simulink model "afe_abc_inv_psm_2mods"  (R2025b)
settings: Solver=ode1be  StartTime=0.0  StopTime=simlength  FixedStep=tc  MaxStep=tc
values from neighbouring files (symbols this model uses):
  n1 = 35    [voltage_islandmode_spectrum_analysis.m]    (also in voltage_spectrum_analysis.m)
undefined symbols (not defined in the file or in its folder): Adrso, afe_pwm_phase_shift_mod1, afe_pwm_phase_shift_mod2, Amplitude_U, Amplitude_V, Amplitude_W, Aresd, Bresd, Cresd, Crso, CTRPIFF_CLIP_RELEASE, dead_time_AFE, dead_time_INV, deepNEGeta, deepNEGxi, deepPOSxi, emf_fb_p, emf_fb_p_ccaller_1, emf_fb_p_ccaller_2, emf_p, emf_p_ccaller_1, emf_p_ccaller_2, end_time_LVRT, fPWM_AFE, fPWM_INV, g0_161Hz, g0_500Hz, g1_161Hz, g1_500Hz, i_grid_neg_eta_lim, i_grid_neg_eta_red_lim, i_grid_neg_xi_lim, i_grid_neg_xi_red_lim, i_grid_pos_eta_lim, i_grid_pos_eta_red_lim, ibez, id_lim, ieta_neg_ref_lim, ieta_pos_ref_lim, Igrid_phase_normalization_factor, inv_pwm_phase_shift_mod1, iq_lim, ixi_pos_ref_lim, k_frt_ref, kg, ki_afe, ki_i, ki_rc_neg_grid, ki_rc_pos_grid, ki_vs, ki_w, kp_afe, kp_i, kp_rc_neg_grid, kp_rc_pos_grid, kp_vs, kp_w, kw, l1, l2 ... (+55)
libraries: fl_lib x215, nesl_utility x107, simulink x22, cstblocks x18, threephase_inductor_lib x4, single_phase_transformer_lib x3, flexshaft_lib x1, psm x1
(part 10 of 17)

== system afe_abc_inv_psm_2mods/afe_abc_inv_psm_mod1/AFE_control/afe_control/grid_voltage_phase_lock_loops/dq_pll_ccaller/first_harmonic_tracker_phase_w ==
  u : Inport
  Bus Selector : BusSelector  OutputSignals=output_pu_hat
  C Caller : CCaller  FunctionName=first_harmonic_tracker_process_simulink  PortSpecificationStruct="%)30     .    V @   8    (     @         %    \"     4    !     0         %  0 \"0    $    _    07)G3F%M90  4&]R=$YA;64 4V-O<&4     26YD97@     5'EP90      4VEZ90      27-';&]B86P   X    P    !@    @    $          4    (     0    ,    !         !   P!O=70 #@   #     &    \"     0         !0    @    !     P    $         $  # &]U=  .    .     8    (    !          %    \"     $    &     0         0   ...(+2669 chars)"
  Constant : Constant  Value=ts_afe
  Constant1 : Constant  Value=4
  Data Type Conversion1 : DataTypeConversion  OutDataTypeStr=single  SaturateOnIntegerOverflow=off  RndMeth=Floor
  Data Type Conversion2 : DataTypeConversion  OutDataTypeStr=single  SaturateOnIntegerOverflow=off  RndMeth=Floor
  Data Type Conversion3 : DataTypeConversion  OutDataTypeStr=uint8  SaturateOnIntegerOverflow=off  RndMeth=Floor
  Data Type Conversion4 : DataTypeConversion  OutDataTypeStr=double  SaturateOnIntegerOverflow=off  RndMeth=Floor
  Data Type Conversion5 : DataTypeConversion  OutDataTypeStr=uint8  SaturateOnIntegerOverflow=off  RndMeth=Floor
  Step : Step  Time=0.0125  Before=1  After=0
  u_hat : Outport
  wires:
  Data Type Conversion4/1 -> u_hat/1
  Data Type Conversion3/1 -> C Caller/1
  Data Type Conversion1/1 -> C Caller/3
  Data Type Conversion2/1 -> C Caller/2
  C Caller/1 -> Bus Selector/1
  Bus Selector/1 -> Data Type Conversion4/1  "<output_pu_hat>"
  Step/1 -> Data Type Conversion3/1
  u/1 -> Data Type Conversion2/1
  Constant/1 -> Data Type Conversion1/1
  Data Type Conversion5/1 -> C Caller/4
  Constant1/1 -> Data Type Conversion5/1

== system afe_abc_inv_psm_2mods/afe_abc_inv_psm_mod1/AFE_control/afe_control/grid_voltage_sequences/voltage_sequence_avg/average_filter_ccaller ==
  v_grid_pos_xi : Inport
  v_grid_pos_eta : Inport  Port=2
  v_grid_neg_xi : Inport  Port=3
  v_grid_neg_eta : Inport  Port=4
  Moving Average Filter1 : Subsystem
  Moving Average Filter2 : Subsystem
  Moving Average Filter3 : Subsystem
  Moving Average Filter4 : Subsystem
  v_grid_pos_xi_avg : Outport
  v_grid_pos_eta_avg : Outport  Port=2
  v_grid_neg_xi_avg : Outport  Port=3
  v_grid_neg_eta_avg : Outport  Port=4
  wires:
  Moving Average Filter2/1(xi) -> v_grid_pos_eta_avg/1
  [omega_grid_pll_mod1] -> Moving Average Filter1/2(In3), Moving Average Filter2/2(In3), Moving Average Filter4/2(In3), Moving Average Filter3/2(In3)
  v_grid_pos_xi/1 -> Moving Average Filter1/1(In2)
  v_grid_neg_xi/1 -> Moving Average Filter3/1(In2)
  v_grid_neg_eta/1 -> Moving Average Filter4/1(In2)
  Moving Average Filter3/1(xi) -> v_grid_neg_xi_avg/1
  Moving Average Filter4/1(xi) -> v_grid_neg_eta_avg/1
  Moving Average Filter1/1(xi) -> v_grid_pos_xi_avg/1
  v_grid_pos_eta/1 -> Moving Average Filter2/1(In2)

== system afe_abc_inv_psm_2mods/afe_abc_inv_psm_mod1/AFE_control/afe_control/grid_voltage_sequences/voltage_sequence_avg/average_filter_simulink ==
  v_grid_pos_xi : Inport
  v_grid_pos_eta : Inport  Port=2
  v_grid_neg_xi : Inport  Port=3
  v_grid_neg_eta : Inport  Port=4
  moving_avarage_1 : Subsystem
  moving_avarage_2 : Subsystem
  moving_avarage_3 : Subsystem
  moving_avarage_4 : Subsystem
  v_grid_pos_xi_avg : Outport
  v_grid_pos_eta_avg : Outport  Port=2
  v_grid_neg_xi_avg : Outport  Port=3
  v_grid_neg_eta_avg : Outport  Port=4
  wires:
  v_grid_neg_xi/1 -> moving_avarage_3/1(u)
  v_grid_pos_xi/1 -> moving_avarage_1/1(u)
  v_grid_neg_eta/1 -> moving_avarage_4/1(u)
  v_grid_pos_eta/1 -> moving_avarage_2/1(u)
  moving_avarage_1/1(y) -> v_grid_pos_xi_avg/1  "v_grid_pos_xi_avg"
  moving_avarage_2/1(y) -> v_grid_pos_eta_avg/1  "v_grid_pos_eta_avg"
  moving_avarage_3/1(y) -> v_grid_neg_xi_avg/1  "v_grid_neg_xi_avg"
  moving_avarage_4/1(y) -> v_grid_neg_eta_avg/1  "v_grid_neg_eta_avg"

== system afe_abc_inv_psm_2mods/afe_abc_inv_psm_mod1/INV_control/inverter_control/current_ctrl/bemf_observer/bemf_observer ==
  ialpha_pu : Inport
  ibeta_pu : Inport  Port=2
  ualpha_pu : Inport  Port=3
  ubeta_pu : Inport  Port=4
  udc_pu : Inport  Port=5
  Gain : Gain  Gain=psi_m_norm
  Gain1 : Gain  Gain=psi_m_norm
  Trigonometric Function : Trigonometry  Operator=cos
  Trigonometric Function1 : Trigonometry
  double_integrator_observer : Subsystem
  psi_alpha_hat : Subsystem
  psi_beta_hat : Subsystem
  theta_bemf_hat : Subsystem
  omega_pu : Outport
  theta_hat : Outport  Port=2
  tag scope: psi_r_alpha_hat_mod1=global, psi_r_alpha_pu_hat_mod1=global, psi_r_beta_hat_mod1=global, psi_r_beta_pu_hat_mod1=global, psi_r_m_alpha_mod1=global, psi_r_m_beta_mod1=global, theta_bemf_hat_mod1=global
  wires:
  Trigonometric Function/1 -> Gain/1
  Trigonometric Function1/1 -> Gain1/1
  ialpha_pu/1 -> psi_alpha_hat/2(ialpha)
  ibeta_pu/1 -> psi_beta_hat/2(ibeta)
  psi_alpha_hat/2(psi_r_alpha_hat) -> [psi_r_alpha_hat_mod1]
  psi_beta_hat/2(psi_r_beta_hat) -> [psi_r_beta_hat_mod1]
  [psi_r_alpha_hat_mod1] -> theta_bemf_hat/1(psi_r_alpha_hat)
  [psi_r_beta_hat_mod1] -> theta_bemf_hat/2(psi_r_beta_hat)
  ualpha_pu/1 -> psi_alpha_hat/1(ualpha)
  ubeta_pu/1 -> psi_beta_hat/1(ubeta)
  [theta_hat_mod1] -> Trigonometric Function/1, Trigonometric Function1/1
  Gain/1 -> [psi_r_m_alpha_mod1]
  Gain1/1 -> [psi_r_m_beta_mod1]
  theta_bemf_hat/1(theta_emf_hat) -> [theta_bemf_hat_mod1]
  [theta_bemf_hat_mod1] -> double_integrator_observer/1(theta)
  double_integrator_observer/1(omega_pu_hat) -> omega_pu/1
  double_integrator_observer/2(theta_hat) -> theta_hat/1
  [psi_r_alpha_hat_mod1] -> [psi_r_alpha_pu_hat_mod1]
  [psi_r_beta_hat_mod1] -> [psi_r_beta_pu_hat_mod1]
  udc_pu/1 -> psi_beta_hat/3(udc), psi_alpha_hat/3(udc)

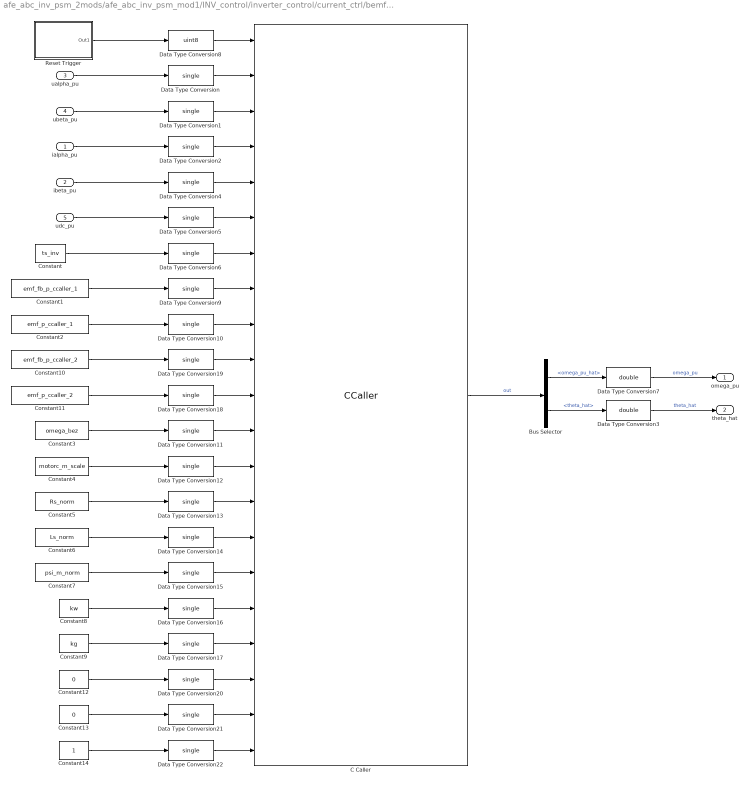
== system afe_abc_inv_psm_2mods/afe_abc_inv_psm_mod1/INV_control/inverter_control/current_ctrl/bemf_observer/bemf_observer_ccaller ==
  ialpha_pu : Inport
  ibeta_pu : Inport  Port=2
  ualpha_pu : Inport  Port=3
  ubeta_pu : Inport  Port=4
  udc_pu : Inport  Port=5
  Bus Selector : BusSelector  OutputSignals=omega_pu_hat,theta_hat
  C Caller : CCaller  FunctionName=bemf_obsv_process_simulink  PortSpecificationStruct="%)30     .    N\"8   8    (     @         %    \"    !8    !     0         %  0 \"0    $    _    07)G3F%M90  4&]R=$YA;64 4V-O<&4     26YD97@     5'EP90      4VEZ90      27-';&]B86P   X    P    !@    @    $          4    (     0    ,    !         !   P!O=70 #@   #     &    \"     0         !0    @    !     P    $         $  # &]U=  .    .     8    (    !          %    \"     $    &     0         0  ...(+12985 chars)"
  Constant : Constant  Value=ts_inv
  Constant1 : Constant  Value=emf_fb_p_ccaller_1
  Constant10 : Constant  Value=emf_fb_p_ccaller_2
  Constant11 : Constant  Value=emf_p_ccaller_2
  Constant12 : Constant  Value=0
  Constant13 : Constant  Value=0
  Constant14 : Constant
  Constant2 : Constant  Value=emf_p_ccaller_1
  Constant3 : Constant  Value=omega_bez
  Constant4 : Constant  Value=motorc_m_scale
  Constant5 : Constant  Value=Rs_norm
  Constant6 : Constant  Value=Ls_norm
  Constant7 : Constant  Value=psi_m_norm
  Constant8 : Constant  Value=kw
  Constant9 : Constant  Value=kg
  Data Type Conversion{,1..2,4..6,9..22} (20 alike) : DataTypeConversion  OutDataTypeStr=single  SaturateOnIntegerOverflow=off  RndMeth=Floor
  Data Type Conversion3 : DataTypeConversion  OutDataTypeStr=double  SaturateOnIntegerOverflow=off  RndMeth=Floor
  Data Type Conversion7 : DataTypeConversion  OutDataTypeStr=double  SaturateOnIntegerOverflow=off  RndMeth=Floor
  Data Type Conversion8 : DataTypeConversion  OutDataTypeStr=uint8  SaturateOnIntegerOverflow=off  RndMeth=Floor
  Reset Trigger : Subsystem
  omega_pu : Outport
  theta_hat : Outport  Port=2
  wires:
  Data Type Conversion5/1 -> C Caller/6
  Data Type Conversion/1 -> C Caller/2
  C Caller/1 -> Bus Selector/1  "out"
  Data Type Conversion1/1 -> C Caller/3
  Data Type Conversion4/1 -> C Caller/5
  Data Type Conversion2/1 -> C Caller/4
  Data Type Conversion6/1 -> C Caller/7
  Bus Selector/2 -> Data Type Conversion3/1  "<theta_hat>"
  Bus Selector/1 -> Data Type Conversion7/1  "<omega_pu_hat>"
  Data Type Conversion7/1 -> omega_pu/1  "omega_pu"
  Data Type Conversion3/1 -> theta_hat/1  "theta_hat"
  Data Type Conversion8/1 -> C Caller/1
  Data Type Conversion9/1 -> C Caller/8
  Data Type Conversion10/1 -> C Caller/9
  Data Type Conversion19/1 -> C Caller/10
  Data Type Conversion18/1 -> C Caller/11
  Data Type Conversion11/1 -> C Caller/12
  Data Type Conversion12/1 -> C Caller/13
  Data Type Conversion13/1 -> C Caller/14
  Data Type Conversion14/1 -> C Caller/15
  Data Type Conversion15/1 -> C Caller/16
  Data Type Conversion16/1 -> C Caller/17
  Data Type Conversion17/1 -> C Caller/18
  Data Type Conversion20/1 -> C Caller/19
  Data Type Conversion21/1 -> C Caller/20
  Data Type Conversion22/1 -> C Caller/21
  Constant14/1 -> Data Type Conversion22/1
  Constant13/1 -> Data Type Conversion21/1
  Constant12/1 -> Data Type Conversion20/1
  Constant9/1 -> Data Type Conversion17/1
  Constant8/1 -> Data Type Conversion16/1
  Constant7/1 -> Data Type Conversion15/1
  Constant6/1 -> Data Type Conversion14/1
  Constant5/1 -> Data Type Conversion13/1
  Constant4/1 -> Data Type Conversion12/1
  Constant3/1 -> Data Type Conversion11/1
  Constant11/1 -> Data Type Conversion18/1
  Constant10/1 -> Data Type Conversion19/1
  Constant2/1 -> Data Type Conversion10/1
  Constant1/1 -> Data Type Conversion9/1
  Constant/1 -> Data Type Conversion6/1
  ibeta_pu/1 -> Data Type Conversion4/1
  ialpha_pu/1 -> Data Type Conversion2/1
  ubeta_pu/1 -> Data Type Conversion1/1
  ualpha_pu/1 -> Data Type Conversion/1
  Reset Trigger/1(Out1) -> Data Type Conversion8/1
  udc_pu/1 -> Data Type Conversion5/1

== system afe_abc_inv_psm_2mods/afe_abc_inv_psm_mod1/INV_control/inverter_control/current_ctrl/bemf_observer/phase_fault ==
  double_integrator_observer : Subsystem
  phase_fault : Subsystem
  omega_pu_encoder : Outport
  theta_hat_encoder : Outport  Port=2
  wires:
  [theta_elec_psm] -> phase_fault/1(theta_pmsm)  "theta_pmsm"
  double_integrator_observer/2(theta_hat) -> theta_hat_encoder/1  "theta_hat_encoder"
  phase_fault/1(theta) -> double_integrator_observer/1(theta)
  double_integrator_observer/1(omega_pu_hat) -> omega_pu_encoder/1  "omega_pu_encoder"

== system afe_abc_inv_psm_2mods/afe_abc_inv_psm_mod1/INV_control/inverter_control/current_ctrl/current_ctrl/MTPA _mod1 ==
  iq_ref : Inport
  Gain1 : Gain  Gain=1/(Ld_norm - Lq_norm)/2
  Gain2 : Gain  Gain=1/(Ld_norm - Lq_norm)/2
  Gain3 : Gain  Gain=-1
  Math Function1 : Math  Operator=magnitude^2  SignedPower=on
  Math Function4 : Math  Operator=magnitude^2  SignedPower=on
  Sqrt : Sqrt
  Sum : Sum  Inputs=|++
  Sum1 : Sum  Inputs=|-+
  id_ref_pu < x < 0 : Saturate  UpperLimit=0  LowerLimit=-id_lim
  Id_ref_mtpa : Outport  VectorParamsAs1DForOutWhenUnconnected=off
  wires:
  Sum1/1 -> Gain3/1
  id_ref_pu < x < 0/1 -> Id_ref_mtpa/1
  Math Function4/1 -> Sum/1
  Math Function1/1 -> Sum/2
  Gain1/1 -> Math Function4/1
  Sum/1 -> Sqrt/1
  Sqrt/1 -> Sum1/2
  iq_ref/1 -> Math Function1/1
  Gain2/1 -> Sum1/1
  [omega_hat_pu_mod1] -> Gain1/1, Gain2/1
  Gain3/1 -> id_ref_pu < x < 0/1

== system afe_abc_inv_psm_2mods/afe_abc_inv_psm_mod1/INV_control/inverter_control/current_ctrl/current_ctrl/dq_pi_with_vector_antiwindup mod1 ==
  id_ref : Inport
  id : Inport  Port=2
  iq_ref : Inport  Port=3
  iq : Inport  Port=4
  udc_pu : Inport  Port=5
  Variant Source : VariantSource  VariantControls={use_current_controller_from_simulink_module_1 == 1, use_current_controller_from_ccaller_module_1 == 1}
  Variant Source1 : VariantSource  VariantControls={use_current_controller_from_simulink_module_1 == 1, use_current_controller_from_ccaller_module_1 == 1}
  dq_vector_pi : Subsystem
  dq_vector_pi_ccaller : Subsystem
  simulink/Ccaller VectorPI : Scope  NumInputPorts=2
      settings: ActiveDisplayYMinimum=-0.12579688616096973  ActiveDisplayYMaximum=0.43534495122730732
  ctrl_d_u : Outport
  ctrl_q_u : Outport  Port=2
  wires:
  id/1 -> dq_vector_pi_ccaller/1(id), dq_vector_pi/1(id)  "id"
  id_ref/1 -> dq_vector_pi_ccaller/2(id_ref), dq_vector_pi/2(id_ref)  "id_ref"
  iq/1 -> dq_vector_pi_ccaller/3(iq), dq_vector_pi/3(iq)  "iq"
  iq_ref/1 -> dq_vector_pi_ccaller/4(iq_ref), dq_vector_pi/4(iq_ref)  "iq_ref"
  dq_vector_pi/1(md_sat) -> Variant Source/1
  dq_vector_pi_ccaller/2(uq_ctrl_out) -> Variant Source1/2
  dq_vector_pi/2(mq_sat) -> Variant Source1/1
  dq_vector_pi_ccaller/1(ud_ctrl_out) -> Variant Source/2
  Variant Source/1 -> ctrl_d_u/1, simulink/Ccaller VectorPI/1  "ctrl_d_u"
  Variant Source1/1 -> simulink/Ccaller VectorPI/2, ctrl_q_u/1  "ctrl_q_u"
  udc_pu/1 -> dq_vector_pi_ccaller/5(udc_pu)

== system afe_abc_inv_psm_2mods/afe_abc_inv_psm_mod1/INV_control/inverter_control/current_ctrl/current_ctrl/id_ref _mod1 ==
  id_mtpa : Inport
  Constant : Constant  Value=0
  Variant Source : VariantSource  VariantControls={use_mtpa == 1, use_mtpa == 0}
  id_ref : Outport
  wires:
  Variant Source/1 -> id_ref/1
  id_mtpa/1 -> Variant Source/1
  Constant/1 -> Variant Source/2

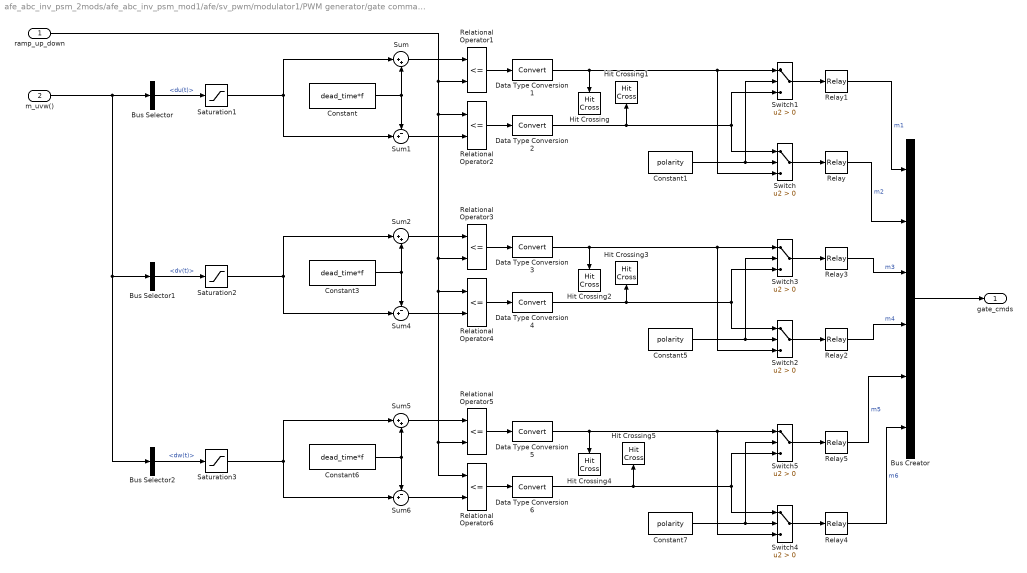
== system afe_abc_inv_psm_2mods/afe_abc_inv_psm_mod1/afe/sv_pwm/modulator1/PWM generator/gate commands ==
  ramp_up_down : Inport
  m_uvw() : Inport  Port=2
  Bus Creator : BusCreator  Inputs=6
  Bus Selector : BusSelector  OutputSignals=du(t)
  Bus Selector1 : BusSelector  OutputSignals=dv(t)
  Bus Selector2 : BusSelector  OutputSignals=dw(t)
  Constant : Constant  Value=dead_time*f
  Constant1 : Constant  Value=polarity
  Constant3 : Constant  Value=dead_time*f
  Constant5 : Constant  Value=polarity
  Constant6 : Constant  Value=dead_time*f
  Constant7 : Constant  Value=polarity
  Data Type Conversion{1..6} (6 alike) : DataTypeConversion
  Hit Crossing{,1..5} (6 alike) : HitCross  ShowOutputPort=off
  Relational Operator{1..6} (6 alike) : RelationalOperator  Operator=<=  InputSameDT=off
  Relay{,1..5} (6 alike) : Relay  OnOutputValue=pos_cmd_gate  OffOutputValue=neg_cmd_gate
  Saturation1 : Saturate  UpperLimit=m_up  LowerLimit=m_low
  Saturation2 : Saturate  UpperLimit=m_up  LowerLimit=m_low
  Saturation3 : Saturate  UpperLimit=m_up  LowerLimit=m_low
  Sum : Sum  Inputs=|++  SaturateOnIntegerOverflow=on
  Sum1 : Sum  Inputs=-+|  SaturateOnIntegerOverflow=on
  Sum2 : Sum  Inputs=|++  SaturateOnIntegerOverflow=on
  Sum4 : Sum  Inputs=-+|  SaturateOnIntegerOverflow=on
  Sum5 : Sum  Inputs=|++  SaturateOnIntegerOverflow=on
  Sum6 : Sum  Inputs=-+|  SaturateOnIntegerOverflow=on
  Switch{,1..5} (6 alike) : Switch  Criteria=u2 > Threshold  SaturateOnIntegerOverflow=off  InputSameDT=off
  gate_cmds : Outport
  wires:
  Data Type Conversion6/1 -> Switch4/1, Switch5/3, Hit Crossing5/1
  Constant1/1 -> Switch1/2, Switch/2
  Data Type Conversion1/1 -> Switch/3, Switch1/1, Hit Crossing/1
  Constant3/1 -> Sum4/1, Sum2/2
  m_uvw()/1 -> Bus Selector2/1, Bus Selector1/1, Bus Selector/1
  Relay4/1 -> Bus Creator/6  "m6"
  Constant6/1 -> Sum5/2, Sum6/1
  Saturation1/1 -> Sum1/2, Sum/1
  Data Type Conversion3/1 -> Switch2/3, Switch3/1, Hit Crossing2/1
  Data Type Conversion2/1 -> Switch/1, Switch1/3, Hit Crossing1/1
  Relational Operator1/1 -> Data Type Conversion1/1
  Bus Creator/1 -> gate_cmds/1
  Data Type Conversion5/1 -> Switch4/3, Switch5/1, Hit Crossing4/1
  Sum1/1 -> Relational Operator2/2
  Constant5/1 -> Switch2/2, Switch3/2
  Switch/1 -> Relay/1
  Sum/1 -> Relational Operator1/1
  Relational Operator6/1 -> Data Type Conversion6/1
  Relay2/1 -> Bus Creator/4  "m4"
  Saturation3/1 -> Sum5/1, Sum6/2
  Constant7/1 -> Switch5/2, Switch4/2
  Sum5/1 -> Relational Operator5/1
  Bus Selector/1 -> Saturation1/1  "<du(t)>"
  Data Type Conversion4/1 -> Switch2/1, Switch3/3, Hit Crossing3/1
  ramp_up_down/1 -> Relational Operator3/2, Relational Operator6/1, Relational Operator5/2, Relational Operator4/1, Relational Operator2/1, Relational Operator1/2
  Switch4/1 -> Relay4/1
  Relational Operator5/1 -> Data Type Conversion5/1
  Switch5/1 -> Relay5/1
  Saturation2/1 -> Sum4/2, Sum2/1
  Relational Operator3/1 -> Data Type Conversion3/1
  Sum2/1 -> Relational Operator3/1
  Switch1/1 -> Relay1/1
  Relay3/1 -> Bus Creator/3  "m3"
  Relational Operator2/1 -> Data Type Conversion2/1
  Bus Selector1/1 -> Saturation2/1  "<dv(t)>"
  Switch3/1 -> Relay3/1
  Sum4/1 -> Relational Operator4/2
  Relay/1 -> Bus Creator/2  "m2"
  Relational Operator4/1 -> Data Type Conversion4/1
  Bus Selector2/1 -> Saturation3/1  "<dw(t)>"
  Relay1/1 -> Bus Creator/1  "m1"
  Sum6/1 -> Relational Operator6/2
  Constant/1 -> Sum/2, Sum1/1
  Relay5/1 -> Bus Creator/5  "m5"
  Switch2/1 -> Relay2/1

== system afe_abc_inv_psm_2mods/afe_abc_inv_psm_mod1/inverter/inverter/sv_pwm/modulator1/PWM generator ==
  time_source : Inport
  phase : Inport  Port=2
  m_uvw() : Inport  Port=3
  Constant8 : Constant  Value=tc
  Constant9 : Constant  Value=f
  MATLAB Function : MATLAB Function  TreatAsAtomicUnit=on  SystemSampleTime=tc
  MATLAB Function1 : MATLAB Function  TreatAsAtomicUnit=on  SystemSampleTime=tc
  gate commands : Subsystem
  period : Constant  Value=1/f
  trgo : Outport
  gate_cmds : Outport  Port=2
  wires:
  period/1 -> MATLAB Function/3(period)
  phase/1 -> MATLAB Function/2(phase)
  MATLAB Function/1(y) -> gate commands/1(ramp_up_down), MATLAB Function1/3(ramp_up_down)
  MATLAB Function1/1(trgo) -> trgo/1
  Constant8/1 -> MATLAB Function1/1(sampling_time)
  Constant9/1 -> MATLAB Function1/2(fPWM)
  m_uvw()/1 -> gate commands/2(m_uvw())
  gate commands/1(gate_cmds) -> gate_cmds/1
  time_source/1 -> MATLAB Function/1(t)

== system afe_abc_inv_psm_2mods/afe_abc_inv_psm_mod2/AFE_control/afe_control/FRT-VDE4110/FRT-Detection/dvxi_n//dt ==
  x : Inport
  Gain : Gain  Gain=l1
  Gain1 : Gain  Gain=l2
  Gain5 : Gain  Gain=ts_afe
  Sum : Sum  Inputs=-+|
  Sum1 : Sum  Inputs=|++
  Sum2 : Sum  Inputs=|++
  Sum8 : Sum  Inputs=++|
  Unit Delay1 : UnitDelay  SampleTime=-1  HasFrameUpgradeWarning=on
  Unit Delay2 : UnitDelay  SampleTime=-1  HasFrameUpgradeWarning=on
  xdot_hat : Outport  VectorParamsAs1DForOutWhenUnconnected=off
  wires:
  Gain1/1 -> Sum2/1
  x/1 -> Sum/2  "x"
  Gain5/1 -> Sum8/1
  Sum1/1 -> Unit Delay2/1
  Gain/1 -> Sum1/1
  Unit Delay2/1 -> xdot_hat/1, Sum1/2, Gain5/1
  Sum2/1 -> Sum8/2
  Unit Delay1/1 -> Sum2/2, Sum/1  "x_hat"
  Sum/1 -> Gain1/1, Gain/1
  Sum8/1 -> Unit Delay1/1

== system afe_abc_inv_psm_2mods/afe_abc_inv_psm_mod2/AFE_control/afe_control/FRT-VDE4110/FRT-Detection/dvxi_p//dt ==
  x : Inport
  Gain : Gain  Gain=l1
  Gain1 : Gain  Gain=l2
  Gain5 : Gain  Gain=ts_afe
  Sum : Sum  Inputs=-+|
  Sum1 : Sum  Inputs=|++
  Sum2 : Sum  Inputs=|++
  Sum8 : Sum  Inputs=++|
  Unit Delay1 : UnitDelay  SampleTime=-1  HasFrameUpgradeWarning=on
  Unit Delay2 : UnitDelay  SampleTime=-1  HasFrameUpgradeWarning=on
  xdot_hat : Outport  VectorParamsAs1DForOutWhenUnconnected=off
  wires:
  Unit Delay2/1 -> Gain5/1, Sum1/2, xdot_hat/1
  Sum8/1 -> Unit Delay1/1
  Sum/1 -> Gain/1, Gain1/1
  Unit Delay1/1 -> Sum/1, Sum2/2  "x_hat"
  Sum2/1 -> Sum8/2
  Gain/1 -> Sum1/1
  Sum1/1 -> Unit Delay2/1
  Gain5/1 -> Sum8/1
  x/1 -> Sum/2  "x"
  Gain1/1 -> Sum2/1

== system afe_abc_inv_psm_2mods/afe_abc_inv_psm_mod2/AFE_control/afe_control/FRT-VDE4110/FRT-PosNegReactiveCurrentReferences/avg_flt_500ms ==
  In1 : Inport
  Constant : Constant  Value=2*pi/500e-3
  Constant1 : Constant  Value=ts_afe
  Constant2 : Constant
  Sum : Sum  Inputs=|-+
  avg_flt_1 : MATLAB Function  TreatAsAtomicUnit=on
  Out1 : Outport  VectorParamsAs1DForOutWhenUnconnected=off
  wires:
  Sum/1 -> avg_flt_1/4(enable)
  [frt_active_mod2] -> Sum/1
  Constant2/1 -> Sum/2
  In1/1 -> avg_flt_1/1(x)  "input"
  Constant/1 -> avg_flt_1/2(w)
  Constant1/1 -> avg_flt_1/3(ts)
  avg_flt_1/1(y1) -> Out1/1  "output"

== system afe_abc_inv_psm_2mods/afe_abc_inv_psm_mod2/AFE_control/afe_control/FRT-VDE4110/FRT-PosNegReactiveCurrentReferences/avg_flt_500ms1 ==
  In1 : Inport
  Constant : Constant  Value=2*pi/500e-3
  Constant1 : Constant  Value=ts_afe
  Constant2 : Constant
  Sum : Sum  Inputs=|-+
  avg_flt_1 : MATLAB Function  TreatAsAtomicUnit=on
  Out1 : Outport  VectorParamsAs1DForOutWhenUnconnected=off
  wires:
  avg_flt_1/1(y1) -> Out1/1  "output"
  Constant1/1 -> avg_flt_1/3(ts)
  Constant/1 -> avg_flt_1/2(w)
  In1/1 -> avg_flt_1/1(x)  "input"
  Constant2/1 -> Sum/2
  [frt_active_mod2] -> Sum/1
  Sum/1 -> avg_flt_1/4(enable)

== system afe_abc_inv_psm_2mods/afe_abc_inv_psm_mod2/AFE_control/afe_control/FRT-VDE4110/FRT-PosNegReactiveCurrentReferences/avg_flt_500ms2 ==
  In1 : Inport
  Constant : Constant  Value=2*pi/500e-3
  Constant1 : Constant  Value=ts_afe
  Constant2 : Constant
  Sum : Sum  Inputs=|-+
  avg_flt_1 : MATLAB Function  TreatAsAtomicUnit=on
  Out1 : Outport  VectorParamsAs1DForOutWhenUnconnected=off
  wires:
  Sum/1 -> avg_flt_1/4(enable)
  [frt_active_mod2] -> Sum/1
  Constant2/1 -> Sum/2
  In1/1 -> avg_flt_1/1(x)  "input"
  Constant/1 -> avg_flt_1/2(w)
  Constant1/1 -> avg_flt_1/3(ts)
  avg_flt_1/1(y1) -> Out1/1  "output"

== system afe_abc_inv_psm_2mods/afe_abc_inv_psm_mod2/AFE_control/afe_control/FRT-VDE4110/FRT-PosNegReactiveCurrentReferences/avg_flt_500ms3 ==
  In1 : Inport
  Constant : Constant  Value=2*pi/500e-3
  Constant1 : Constant  Value=ts_afe
  Constant2 : Constant
  Sum : Sum  Inputs=|-+
  avg_flt_1 : MATLAB Function  TreatAsAtomicUnit=on
  Out1 : Outport  VectorParamsAs1DForOutWhenUnconnected=off
  wires:
  avg_flt_1/1(y1) -> Out1/1  "output"
  Constant1/1 -> avg_flt_1/3(ts)
  Constant/1 -> avg_flt_1/2(w)
  In1/1 -> avg_flt_1/1(x)  "input"
  Constant2/1 -> Sum/2
  [frt_active_mod2] -> Sum/1
  Sum/1 -> avg_flt_1/4(enable)

== system afe_abc_inv_psm_2mods/afe_abc_inv_psm_mod2/AFE_control/afe_control/FRT-VDE4110/FRT-PosNegReactiveCurrentReferences/u_161Hz_flt1 ==
  input : Inport
  Gain3 : Gain  Gain=g1_161Hz
  Gain6 : Gain  Gain=g0_161Hz
  Sum : Sum  Inputs=|++
  Unit Delay1 : UnitDelay  SampleTime=-1  HasFrameUpgradeWarning=on
  output : Outport  VectorParamsAs1DForOutWhenUnconnected=off
  wires:
  Sum/1 -> output/1, Unit Delay1/1
  Gain3/1 -> Sum/2
  Unit Delay1/1 -> Gain3/1
  input/1 -> Gain6/1
  Gain6/1 -> Sum/1

== system afe_abc_inv_psm_2mods/afe_abc_inv_psm_mod2/AFE_control/afe_control/FRT-VDE4110/FRT-PosNegReactiveCurrentReferences/u_161Hz_flt2 ==
  input : Inport
  Gain3 : Gain  Gain=g1_161Hz
  Gain6 : Gain  Gain=g0_161Hz
  Sum : Sum  Inputs=|++
  Unit Delay1 : UnitDelay  SampleTime=-1  HasFrameUpgradeWarning=on
  output : Outport  VectorParamsAs1DForOutWhenUnconnected=off
  wires:
  Gain6/1 -> Sum/1
  input/1 -> Gain6/1
  Unit Delay1/1 -> Gain3/1
  Gain3/1 -> Sum/2
  Sum/1 -> Unit Delay1/1, output/1

== system afe_abc_inv_psm_2mods/afe_abc_inv_psm_mod2/AFE_control/afe_control/FRT-VDE4110/FRT-PosNegReactiveCurrentReferences/u_161Hz_flt3 ==
  input : Inport
  Gain3 : Gain  Gain=g1_161Hz
  Gain6 : Gain  Gain=g0_161Hz
  Sum : Sum  Inputs=|++
  Unit Delay1 : UnitDelay  SampleTime=-1  HasFrameUpgradeWarning=on
  output : Outport  VectorParamsAs1DForOutWhenUnconnected=off
  wires:
  Sum/1 -> output/1, Unit Delay1/1
  Gain3/1 -> Sum/2
  Unit Delay1/1 -> Gain3/1
  input/1 -> Gain6/1
  Gain6/1 -> Sum/1

== system afe_abc_inv_psm_2mods/afe_abc_inv_psm_mod2/AFE_control/afe_control/current_ctrl/Inner Loop Current Control/Current-Control, Phase a ==
  In1 : Inport
  In2 : Inport  Port=2
  Add : Sum
  Cresd./Tcontrol new1 : Gain  Gain=Cresd  Multiplication=Matrix(K*u)
  Gain : Gain  Gain=kp_afe
  Gain1 : Gain  Gain=ki_afe
  Gain2 : Gain  Gain=Bresd  Multiplication=Matrix(K*u)
  Gain3 : Gain  Gain=Aresd  Multiplication=Matrix(K*u)
  Sum : Sum  Inputs=|+-
  Sum2 : Sum  Inputs=|++  SaturateOnIntegerOverflow=on
  Unit Delay : UnitDelay  InitialCondition=[0 0]  SampleTime=-1  HasFrameUpgradeWarning=on
  Out1 : Outport
  wires:
  Cresd./Tcontrol new1/1 -> Add/2  "y(k)"
  Gain3/1 -> Sum2/2
  Sum2/1 -> Unit Delay/1  "x(k+1)"
  Unit Delay/1 -> Cresd./Tcontrol new1/1, Gain3/1  "x(k)"
  Gain2/1 -> Sum2/1
  Gain1/1 -> Gain2/1  "u(k)"
  Gain/1 -> Add/1
  Sum/1 -> Gain/1, Gain1/1
  Add/1 -> Out1/1  "v_a"
  In2/1 -> Sum/2  "isa"
  In1/1 -> Sum/1  "isa_ref"

== system afe_abc_inv_psm_2mods/afe_abc_inv_psm_mod2/AFE_control/afe_control/current_ctrl/Inner Loop Current Control/Current-Control, Phase b ==
  In1 : Inport
  In2 : Inport  Port=2
  Add : Sum
  Cresd./Tcontrol new1 : Gain  Gain=Cresd  Multiplication=Matrix(K*u)
  Gain : Gain  Gain=kp_afe
  Gain1 : Gain  Gain=ki_afe
  Gain2 : Gain  Gain=Bresd  Multiplication=Matrix(K*u)
  Gain3 : Gain  Gain=Aresd  Multiplication=Matrix(K*u)
  Sum : Sum  Inputs=|+-
  Sum2 : Sum  Inputs=|++  SaturateOnIntegerOverflow=on
  Unit Delay : UnitDelay  InitialCondition=[0 0]  SampleTime=-1  HasFrameUpgradeWarning=on
  Out1 : Outport
  wires:
  In1/1 -> Sum/1  "isb_ref"
  In2/1 -> Sum/2  "isb"
  Add/1 -> Out1/1  "v_a"
  Sum/1 -> Gain1/1, Gain/1
  Gain/1 -> Add/1
  Gain1/1 -> Gain2/1  "u(k)"
  Gain2/1 -> Sum2/1
  Unit Delay/1 -> Gain3/1, Cresd./Tcontrol new1/1  "x(k)"
  Sum2/1 -> Unit Delay/1  "x(k+1)"
  Gain3/1 -> Sum2/2
  Cresd./Tcontrol new1/1 -> Add/2  "y(k)"

== system afe_abc_inv_psm_2mods/afe_abc_inv_psm_mod2/AFE_control/afe_control/current_ctrl/Inner Loop Current Control/Current-Control, Phase c ==
  In1 : Inport
  In2 : Inport  Port=2
  Add : Sum
  Cresd./Tcontrol new1 : Gain  Gain=Cresd  Multiplication=Matrix(K*u)
  Gain : Gain  Gain=kp_afe
  Gain1 : Gain  Gain=ki_afe
  Gain2 : Gain  Gain=Bresd  Multiplication=Matrix(K*u)
  Gain3 : Gain  Gain=Aresd  Multiplication=Matrix(K*u)
  Sum : Sum  Inputs=|+-
  Sum2 : Sum  Inputs=|++  SaturateOnIntegerOverflow=on
  Unit Delay : UnitDelay  InitialCondition=[0 0]  SampleTime=-1  HasFrameUpgradeWarning=on
  Out1 : Outport
  wires:
  Cresd./Tcontrol new1/1 -> Add/2  "y(k)"
  Gain3/1 -> Sum2/2
  Sum2/1 -> Unit Delay/1  "x(k+1)"
  Unit Delay/1 -> Cresd./Tcontrol new1/1, Gain3/1  "x(k)"
  Gain2/1 -> Sum2/1
  Gain1/1 -> Gain2/1  "u(k)"
  Gain/1 -> Add/1
  Sum/1 -> Gain/1, Gain1/1
  Add/1 -> Out1/1  "v_a"
  In2/1 -> Sum/2  "isc"
  In1/1 -> Sum/1  "isc_ref"

== system afe_abc_inv_psm_2mods/afe_abc_inv_psm_mod2/AFE_control/afe_control/grid_current_sequences_and_reactive_pwr_ctrl/current_sequence_avg/average_filter_ccaller ==
  i_grid_pos_xi : Inport
  i_grid_pos_eta : Inport  Port=2
  i_grid_neg_xi : Inport  Port=3
  i_grid_neg_eta : Inport  Port=4
  Moving Average Filter1 : Subsystem
  Moving Average Filter2 : Subsystem
  Moving Average Filter3 : Subsystem
  Moving Average Filter5 : Subsystem
  i_grid_pos_xi_avg : Outport
  i_grid_pos_eta_avg : Outport  Port=2
  i_grid_neg_xi_avg : Outport  Port=3
  i_grid_neg_eta_avg : Outport  Port=4
  wires:
  Moving Average Filter5/1(xi) -> i_grid_pos_xi_avg/1
  i_grid_neg_eta/1 -> Moving Average Filter3/1(In2)
  i_grid_pos_xi/1 -> Moving Average Filter5/1(In2)
  Moving Average Filter2/1(xi) -> i_grid_neg_xi_avg/1
  i_grid_neg_xi/1 -> Moving Average Filter2/1(In2)
  Moving Average Filter3/1(xi) -> i_grid_neg_eta_avg/1
  i_grid_pos_eta/1 -> Moving Average Filter1/1(In2)
  [omega_grid_pll_mod2] -> Moving Average Filter2/2(In3), Moving Average Filter3/2(In3), Moving Average Filter1/2(In3), Moving Average Filter5/2(In3)
  Moving Average Filter1/1(xi) -> i_grid_pos_eta_avg/1

== system afe_abc_inv_psm_2mods/afe_abc_inv_psm_mod2/AFE_control/afe_control/grid_current_sequences_and_reactive_pwr_ctrl/current_sequence_avg/average_filter_simulink ==
  i_grid_pos_xi : Inport
  i_grid_pos_eta : Inport  Port=2
  i_grid_neg_xi : Inport  Port=3
  i_grid_neg_eta : Inport  Port=4
  moving_avarage_1 : Subsystem
  moving_avarage_2 : Subsystem
  moving_avarage_3 : Subsystem
  moving_avarage_4 : Subsystem
  i_grid_pos_xi_avg : Outport
  i_grid_pos_eta_avg : Outport  Port=2
  i_grid_neg_xi_avg : Outport  Port=3
  i_grid_neg_eta_avg : Outport  Port=4
  wires:
  moving_avarage_4/1(y) -> i_grid_neg_eta_avg/1  "i_grid_neg_eta_avg"
  moving_avarage_3/1(y) -> i_grid_neg_xi_avg/1  "i_grid_neg_xi_avg"
  moving_avarage_2/1(y) -> i_grid_pos_eta_avg/1  "i_grid_pos_eta_avg"
  moving_avarage_1/1(y) -> i_grid_pos_xi_avg/1  "i_grid_pos_xi_avg"
  i_grid_neg_eta/1 -> moving_avarage_4/1(u)
  i_grid_neg_xi/1 -> moving_avarage_3/1(u)
  i_grid_pos_eta/1 -> moving_avarage_2/1(u)
  i_grid_pos_xi/1 -> moving_avarage_1/1(u)

== system afe_abc_inv_psm_2mods/afe_abc_inv_psm_mod2/AFE_control/afe_control/grid_current_sequences_and_reactive_pwr_ctrl/sequences_current_control/Negative-Seq. eta-Control ==
  ff : Inport
  e : Inport  Port=2
  1/Ti : Gain  Gain=kp_rc_neg_grid  SaturateOnIntegerOverflow=on  OutDataTypeStr=Inherit: Same as input  ParamDataTypeStr=Inherit: Same as input
  Saturation : Saturate  UpperLimit=ieta_neg_ref_lim  LowerLimit=-ieta_neg_ref_lim
  Sum : Sum  Inputs=|++
  Sum2 : Sum  Inputs=+++  SaturateOnIntegerOverflow=on
  Sum3 : Sum  Inputs=-+  SaturateOnIntegerOverflow=on
  Unit Delay4 : UnitDelay  SampleTime=-1  HasFrameUpgradeWarning=on
  kp : Gain  Gain=ki_rc_neg_grid*ts_afe  SaturateOnIntegerOverflow=on  OutDataTypeStr=Inherit: Same as input  ParamDataTypeStr=Inherit: Same as input
  u : Outport  VectorParamsAs1DForOutWhenUnconnected=off
  wires:
  ff/1 -> Sum/2
  e/1 -> kp/1, 1/Ti/1  "e"
  Sum/1 -> u/1
  Saturation/1 -> Sum3/2, Sum/1
  1/Ti/1 -> Sum3/1, Sum2/1
  Sum2/1 -> Saturation/1
  kp/1 -> Sum2/2
  Sum3/1 -> Unit Delay4/1
  Unit Delay4/1 -> Sum2/3

== system afe_abc_inv_psm_2mods/afe_abc_inv_psm_mod2/AFE_control/afe_control/grid_current_sequences_and_reactive_pwr_ctrl/sequences_current_control/Negative-Seq. xi-Control ==
  ff : Inport
  e : Inport  Port=2
  1/Ti : Gain  Gain=kp_rc_neg_grid  SaturateOnIntegerOverflow=on  OutDataTypeStr=Inherit: Same as input  ParamDataTypeStr=Inherit: Same as input
  Saturation : Saturate  UpperLimit=ieta_pos_ref_lim  LowerLimit=-ieta_pos_ref_lim
  Sum : Sum  Inputs=|++
  Sum2 : Sum  Inputs=+++  SaturateOnIntegerOverflow=on
  Sum3 : Sum  Inputs=-+  SaturateOnIntegerOverflow=on
  Unit Delay4 : UnitDelay  SampleTime=-1  HasFrameUpgradeWarning=on
  kp : Gain  Gain=ki_rc_neg_grid*ts_afe  SaturateOnIntegerOverflow=on  OutDataTypeStr=Inherit: Same as input  ParamDataTypeStr=Inherit: Same as input
  u : Outport  VectorParamsAs1DForOutWhenUnconnected=off
  wires:
  ff/1 -> Sum/2
  e/1 -> kp/1, 1/Ti/1  "e"
  Sum/1 -> u/1
  Saturation/1 -> Sum3/2, Sum/1
  1/Ti/1 -> Sum3/1, Sum2/1
  Sum2/1 -> Saturation/1
  kp/1 -> Sum2/2
  Sum3/1 -> Unit Delay4/1
  Unit Delay4/1 -> Sum2/3

== system afe_abc_inv_psm_2mods/afe_abc_inv_psm_mod2/AFE_control/afe_control/grid_current_sequences_and_reactive_pwr_ctrl/sequences_current_control/Positive-Seq. eta-Control ==
  ff : Inport
  e : Inport  Port=2
  1/Ti : Gain  Gain=kp_rc_pos_grid  SaturateOnIntegerOverflow=on  OutDataTypeStr=Inherit: Same as input  ParamDataTypeStr=Inherit: Same as input
  Saturation : Saturate  UpperLimit=ieta_pos_ref_lim  LowerLimit=-ieta_pos_ref_lim
  Sum : Sum  Inputs=|++
  Sum2 : Sum  Inputs=+++  SaturateOnIntegerOverflow=on
  Sum3 : Sum  Inputs=-+  SaturateOnIntegerOverflow=on
  Unit Delay4 : UnitDelay  SampleTime=-1  HasFrameUpgradeWarning=on
  kp : Gain  Gain=ki_rc_pos_grid*ts_afe  SaturateOnIntegerOverflow=on  OutDataTypeStr=Inherit: Same as input  ParamDataTypeStr=Inherit: Same as input
  u : Outport  VectorParamsAs1DForOutWhenUnconnected=off
  wires:
  ff/1 -> Sum/2
  e/1 -> kp/1, 1/Ti/1  "e"
  Sum/1 -> u/1
  Saturation/1 -> Sum3/2, Sum/1
  1/Ti/1 -> Sum3/1, Sum2/1
  Sum2/1 -> Saturation/1
  kp/1 -> Sum2/2
  Sum3/1 -> Unit Delay4/1
  Unit Delay4/1 -> Sum2/3

== system afe_abc_inv_psm_2mods/afe_abc_inv_psm_mod2/AFE_control/afe_control/grid_voltage_phase_lock_loops/DDSRF-PLL/pll_stageA ==
  gamma_grid : Inport
  ug_abc_pu : Inport  Port=2
  Demux : Demux  Outputs=3
  Math Function : Math  Operator=magnitude^2  SignedPower=on
  Math Function1 : Math  Operator=magnitude^2  SignedPower=on
  Reciprocal Sqrt : Sqrt  Operator=rSqrt
  Saturation : Saturate  UpperLimit=inf  LowerLimit=0.02
  Sum : Sum  Inputs=|++
  mormalization_and_transformation : Subsystem
  sequences : Subsystem
  u_grid_pos_xi : Outport  VectorParamsAs1DForOutWhenUnconnected=off
  u_grid_pos_eta : Outport  Port=2  VectorParamsAs1DForOutWhenUnconnected=off
  tag scope: Vgrid_unorm=global
  wires:
  gamma_grid/1 -> sequences/3(phase_angle)
  sequences/2(u_grid_pos_eta) -> u_grid_pos_eta/1
  sequences/1(u_grid_pos_xi) -> u_grid_pos_xi/1
  ug_abc_pu/1 -> Demux/1
  Demux/1 -> mormalization_and_transformation/1(ug_a)
  Demux/2 -> mormalization_and_transformation/2(ug_b)
  Demux/3 -> mormalization_and_transformation/3(ug_c)
  mormalization_and_transformation/1(ug_alpha) -> Math Function/1, sequences/1(u_grid_alpha)
  mormalization_and_transformation/2(ug_beta) -> Math Function1/1, sequences/2(u_grid_beta)
  Math Function/1 -> Sum/1
  Math Function1/1 -> Sum/2
  Sum/1 -> Saturation/1
  Reciprocal Sqrt/1 -> [Vgrid_unorm]
  Saturation/1 -> Reciprocal Sqrt/1
